simulink model "testemplanner_cs_old"  (R2020a)
settings: Solver=ode5  StartTime=0.0  StopTime=120  FixedStep=1/1000  RelTol=1e-3
PreLoadFcn:
  | mbxruntime.callbacks.PreLoadFcn(bdroot);
PostLoadFcn:
  | mbxruntime.callbacks.PostLoadFcn(bdroot);
InitFcn:
  | mbxruntime.callbacks.InitFcn(bdroot);
StartFcn:
  | mbxruntime.callbacks.StartFcn(bdroot);
StopFcn:
  | mbxruntime.callbacks.StopFcn(bdroot);
model workspace (MAT data in the model file):
  mbox_table : object (value not decoded)
  model_closed = 0
  sim_status = 0
values from neighbouring files (symbols this model uses):
  c_factor = 43.75    [emplanner_init.m]
  cf = -175016    [emplanner_init.m]
  cr = -130634    [emplanner_init.m]
  global_path_x = [0.057304 1.05668625507 2.05480936558 3.05165624935 4.04722112279 5.04150235808 6.03449985569 7.02621407764 8.01664569183 9.00579544113 9.99366409523 10.9802524329 ... (3001 elements, 3001x1)]    [global_path.mat]
  global_path_y = [8.29 8.29 8.29 8.29 8.29 8.29 8.29 8.29 8.29 8.29 8.29 8.29 ... (3001 elements, 3001x1)]    [global_path.mat]
  KD_PID_distance = 0.0    (= 0)    [emplanner_init.m]
  KD_PID_speed = 0    [emplanner_init.m]
  KI_PID_distance = 0.0    (= 0)    [emplanner_init.m]
  KI_PID_speed = 0    [emplanner_init.m]
  KP_PID_distance = 0.5    [emplanner_init.m]
  KP_PID_speed = 1.8    [emplanner_init.m]
  la = 1.265    [emplanner_init.m]
  lb = 2.947-1.265    (= 1.682)    [emplanner_init.m]
  LQR_K1 = k(:,1)'    [emplanner_init.m]
  LQR_K2 = k(:,2)'    [emplanner_init.m]
  LQR_K3 = k(:,3)'    [emplanner_init.m]
  LQR_K4 = k(:,4)'    [emplanner_init.m]
  m = 2020    [emplanner_init.m]
  rack_displacement = [-39.14 , -37.2 , -35.29 , -33.43 , -31.6 , -29.81 , -28.06 , -26.34 , -24.66 ,      -23.01 , -21.38 , -19.79 , -18.23 , -16.69 , -15.18 , -13.7 , -12.23 , -10.8 , -9.38 , -7.98 ,     -6.61 , -5.25 , -3.91 , -2.59 , -1.29 , 0 , 1.27 , 2.54 , 3.78 , 5.02 , 6.24 , 7.46 , 8.66 ,      9.86 , 11.05 , 12.24 , 13.41 , 14.59 , 15.76 , 16.92 , 18.09 , 19.25 , 20.42 , 21.59 , 22.76 ,      23.93 , 25.11 , 26 ...(+26 chars)    [emplanner_init.m]
  right_wheel_ground = [-70 ,-67.2 , -64.4 , -61.6 , -58.8 , -56 , -53.2 , -50.4 , -47.6 , -44.8 , -42 ,      -39.2 , -36.4 , -33.6 , -30.8 , -28 , -25.2 , -22.4 , -19.6 , -16.8 , -14 , -11.2 , -8.4 , -5.6 ,      -2.8 , 0 , 2.8 , 5.6 , 8.4 , 11.2 , 14 , 16.8 , 19.6 , 22.4 , 25.2 , 28 , 30.8 , 33.6 , 36.4 ,      39.2 , 42 , 44.8 , 47.6 , 50.4 , 53.2 , 56 , 58.8 , 61.6 , 64.4 , 67.2 , 70 ]    [emplanner_init.m]
  vx_break_point = zeros(1,5000)    [emplanner_init.m]
undefined symbols (not defined in the file or in its folder): aubr, DiscIntNeverNeededParam, tablebr, vubr
libraries: PreScanSimulinkLibrary x9, Solver_SF x1, simulink_extras x1
(part 4 of 6)

== system testemplanner_cs_old/Audi_A8_Sedan_1/Trajectories/Traj2State1/Traj2State2/Traj2MuxState_Ext ==
  Traj : Inport
  Terminator{1..9} (9 alike) : Terminator
  demux : Subsystem
  x [m] : Outport
  y [m] : Outport  Port=2
  z [m] : Outport  Port=3
  dx [m/s] : Outport  Port=4
  dy [m/s] : Outport  Port=5
  dz [m/s] : Outport  Port=6
  R [rad] : Outport  Port=7
  P [rad] : Outport  Port=8
  Y [rad] : Outport  Port=9
  wires:
  demux/9(Y) -> Y [rad]/1
  demux/7(R) -> R [rad]/1
  demux/5(vely) -> dy [m/s]/1
  demux/4(velx) -> dx [m/s]/1
  demux/10(velR) -> Terminator4/1
  demux/11(velP) -> Terminator5/1
  demux/12(velY) -> Terminator1/1
  demux/13(accx) -> Terminator8/1
  demux/14(accy) -> Terminator9/1
  demux/15(accz) -> Terminator7/1
  demux/18(accY) -> Terminator2/1
  demux/16(accR) -> Terminator3/1
  demux/17(accP) -> Terminator6/1
  demux/3(z) -> z [m]/1
  Traj/1 -> demux/1(traj)
  demux/6(velz) -> dz [m/s]/1
  demux/1(x) -> x [m]/1
  demux/2(y) -> y [m]/1
  demux/8(P) -> P [rad]/1

== system testemplanner_cs_old/Audi_A8_Sedan_1/control module1/control main/longitudinal control double PID/discrete pid ==
  err : Inport
  kp : Inport  Port=2
  ki : Inport  Port=3
  kd : Inport  Port=4
  Add2 : Sum  Inputs=+++
  Add3 : Sum
  Add4 : Sum  Inputs=+-
  Delay3 : Delay  DelayLength=1
  Delay4 : Delay  DelayLength=1
  Divide : Product  Inputs=**
  Divide1 : Product  Inputs=**
  Divide2 : Product  Inputs=**
  Gain : Gain  Gain=0.01
  pid_out : Outport
  wires:
  [KD_PID_distance] -> Divide2/2
  err/1 -> Delay4/1, Divide/2, Add3/1, Add4/1
  Divide/1 -> Add2/1
  Divide2/1 -> Add2/3
  Add3/1 -> Gain/1, Divide1/1
  Delay4/1 -> Add4/2
  [KP_PID_distance] -> Divide/1
  Divide1/1 -> Add2/2
  Delay3/1 -> Add3/2
  [KI_PID_distance] -> Divide1/2
  Add4/1 -> Divide2/1
  Add2/1 -> pid_out/1
  kp/1 -> [KP_PID_distance]
  ki/1 -> [KI_PID_distance]
  kd/1 -> [KD_PID_distance]
  Gain/1 -> Delay3/1

== system testemplanner_cs_old/Audi_A8_Sedan_1/control module1/control main/longitudinal control double PID/discrete pid1 ==
  err : Inport
  kp : Inport  Port=2
  ki : Inport  Port=3
  kd : Inport  Port=4
  Add2 : Sum  Inputs=+++
  Add3 : Sum
  Add4 : Sum  Inputs=+-
  Delay3 : Delay  DelayLength=1
  Delay4 : Delay  DelayLength=1
  Divide : Product  Inputs=**
  Divide1 : Product  Inputs=**
  Divide2 : Product  Inputs=**
  Gain : Gain  Gain=0.01
  pid_out : Outport
  wires:
  Gain/1 -> Delay3/1
  kd/1 -> [KD_PID_distance]
  ki/1 -> [KI_PID_distance]
  kp/1 -> [KP_PID_distance]
  Add2/1 -> pid_out/1
  Add4/1 -> Divide2/1
  [KI_PID_distance] -> Divide1/2
  Delay3/1 -> Add3/2
  Divide1/1 -> Add2/2
  [KP_PID_distance] -> Divide/1
  Delay4/1 -> Add4/2
  Add3/1 -> Divide1/1, Gain/1
  Divide2/1 -> Add2/3
  Divide/1 -> Add2/1
  err/1 -> Add4/1, Add3/1, Divide/2, Delay4/1
  [KD_PID_distance] -> Divide2/2

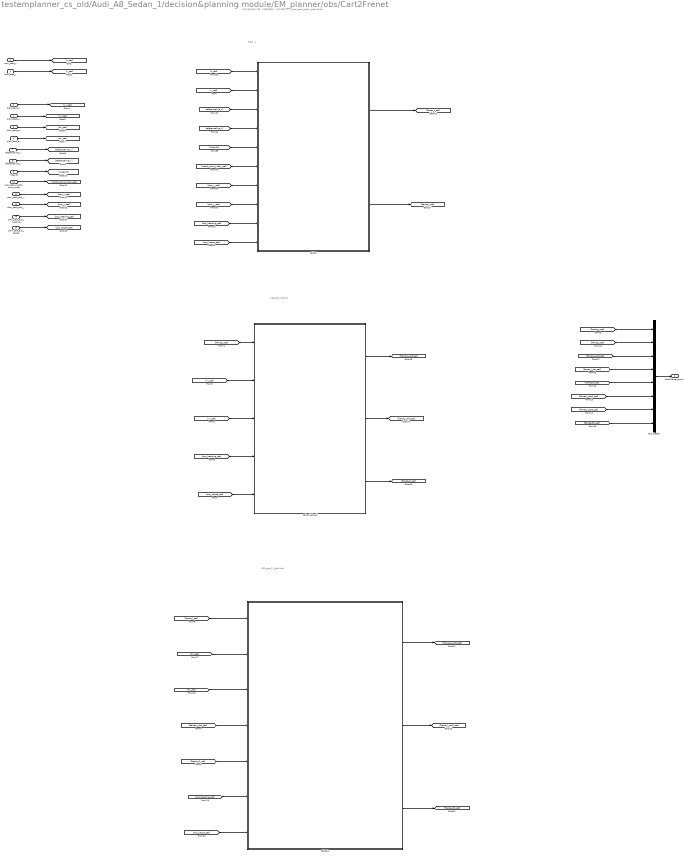
== system testemplanner_cs_old/Audi_A8_Sedan_1/decision&planning module/EM_planner/obs/Cart2Frenet ==
  note: 分成三部分进行计算，方便后续拆分，分别计算S，L，s_dot,l_dot,s_dot2,l_dot2,dl和ddl
  note: 计算S，L
  note: 计算s_dot,l_dot,dl
  note: 计算s_dot_2,l_dot2,ddl
  plan_start_x : Inport
  plan_start_y : Inport  Port=2
  plan_start_vx : Inport  Port=3
  plan_start_vy : Inport  Port=4
  plan_start_ax : Inport  Port=5
  plan_start_ay : Inport  Port=6
  referenceline_x : Inport  Port=7
  referenceline_y : Inport  Port=8
  index2s : Inport  Port=9
  plan_start_match_point_index : Inport  Port=10
  plan_start_proj_x : Inport  Port=11
  plan_start_proj_y : Inport  Port=12
  plan_start_proj_heading : Inport  Port=13
  plan_start_proj_kappa : Inport  Port=14
  Bus Creator : BusCreator  Inputs=8
  CalcSL : MATLAB Function  TreatAsAtomicUnit=on
  CalcSL2 : MATLAB Function  TreatAsAtomicUnit=on
  Calcs_l_dot_dl : MATLAB Function  TreatAsAtomicUnit=on
  Cart2Frenet_result : Outport
  wires:
  CalcSL/1(frenet_s_set) -> [frenet_s_set]
  plan_start_x/1 -> [x_set]
  plan_start_y/1 -> [y_set]
  plan_start_vx/1 -> [vx_set]
  plan_start_vy/1 -> [vy_set]
  plan_start_ax/1 -> [ax_set]
  plan_start_ay/1 -> [ay_set]
  referenceline_x/1 -> [referenceline_x]
  referenceline_y/1 -> [referenceline_y]
  index2s/1 -> [index2s]
  plan_start_match_point_index/1 -> [match_point_index_set]
  plan_start_proj_x/1 -> [proj_x_set]
  plan_start_proj_y/1 -> [proj_y_set]
  plan_start_proj_heading/1 -> [proj_heading_set]
  plan_start_proj_kappa/1 -> [proj_kappa_set]
  [x_set] -> CalcSL/1(x_set)
  [y_set] -> CalcSL/2(y_set)
  [referenceline_x] -> CalcSL/3(referenceline_x)
  [referenceline_y] -> CalcSL/4(referenceline_y)
  [index2s] -> CalcSL/5(index2s)
  [match_point_index_set] -> CalcSL/6(plan_start_match_point_index)
  [proj_x_set] -> CalcSL/7(plan_start_proj_x)
  [proj_y_set] -> CalcSL/8(plan_start_proj_y)
  [proj_heading_set] -> CalcSL/9(plan_start_proj_heading)
  [proj_kappa_set] -> CalcSL/10(plan_start_proj_kappa)
  [proj_kappa_set] -> Calcs_l_dot_dl/5(plan_start_proj_kappa)
  [proj_heading_set] -> Calcs_l_dot_dl/4(plan_start_proj_heading)
  [vx_set] -> Calcs_l_dot_dl/2(vx_set)
  [proj_heading_set] -> CalcSL2/6(plan_start_proj_heading)
  [proj_kappa_set] -> CalcSL2/7(plan_start_proj_kappa)
  CalcSL/2(frenet_l_set) -> [frenet_l_set]
  [frenet_l_set] -> Calcs_l_dot_dl/1(frenet_l_set)
  [vy_set] -> Calcs_l_dot_dl/3(vy_set)
  Calcs_l_dot_dl/1(s_dot_set) -> [frenet_s_dot_set]
  Calcs_l_dot_dl/2(l_dot_set) -> [frenet_l_dot_set]
  Calcs_l_dot_dl/3(dl_set) -> [frenet_dl_set]
  [ax_set] -> CalcSL2/2(ax_set)
  [ay_set] -> CalcSL2/3(ay_set)
  [frenet_dl_set] -> CalcSL2/5(dl_set)
  [frenet_l_set] -> CalcSL2/1(frenet_l_set)
  [frenet_s_dot_set] -> CalcSL2/4(s_dot_set)
  CalcSL2/3(ddl_set) -> [frenet_ddl_set]
  CalcSL2/2(l_dot2_set) -> [frenet_l_dot2_set]
  CalcSL2/1(s_dot2_set) -> [frenet_s_dot2_set]
  [frenet_s_set] -> Bus Creator/1
  [frenet_l_set] -> Bus Creator/2
  [frenet_s_dot_set] -> Bus Creator/3
  [frenet_l_dot_set] -> Bus Creator/4
  [frenet_dl_set] -> Bus Creator/5
  [frenet_s_dot2_set] -> Bus Creator/6
  [frenet_l_dot2_set] -> Bus Creator/7
  [frenet_ddl_set] -> Bus Creator/8
  Bus Creator/1 -> Cart2Frenet_result/1

== system testemplanner_cs_old/Audi_A8_Sedan_1/Trajectories/Traj2State1/Traj2State2/Traj2MuxState_Ext/demux ==
  traj : Inport
  Demux : Demux  Outputs=18
  x : Outport
  y : Outport  Port=2
  z : Outport  Port=3
  velx : Outport  Port=4
  vely : Outport  Port=5
  velz : Outport  Port=6
  R : Outport  Port=7
  P : Outport  Port=8
  Y : Outport  Port=9
  velR : Outport  Port=10
  velP : Outport  Port=11
  velY : Outport  Port=12
  accx : Outport  Port=13
  accy : Outport  Port=14
  accz : Outport  Port=15
  accR : Outport  Port=16
  accP : Outport  Port=17
  accY : Outport  Port=18
  wires:
  Demux/18 -> accY/1
  Demux/17 -> accP/1
  Demux/16 -> accR/1
  Demux/15 -> accz/1
  Demux/14 -> accy/1
  Demux/13 -> accx/1
  Demux/12 -> velY/1
  Demux/11 -> velP/1
  Demux/10 -> velR/1
  Demux/9 -> velz/1
  Demux/8 -> vely/1
  Demux/7 -> velx/1
  Demux/6 -> Y/1
  Demux/5 -> P/1
  traj/1 -> Demux/1
  Demux/4 -> R/1
  Demux/3 -> z/1
  Demux/2 -> y/1
  Demux/1 -> x/1

== matlab function testemplanner_cs_old/Audi_A8_Sedan_1/decision&planning module/EM_planner/Cart2Frenet/CalcSL ==
  data: x_set input; y_set input; referenceline_x input; referenceline_y input; index2s input; plan_start_match_point_index input; plan_start_proj_x input; plan_start_proj_y input; plan_start_proj_heading input; plan_start_proj_kappa input; frenet_s_set output; frenet_l_set output
function [frenet_s_set,frenet_l_set] =fcn(x_set,y_set,referenceline_x,referenceline_y,index2s,plan_start_match_point_index,plan_start_proj_x,plan_start_proj_y,plan_start_proj_heading,plan_start_proj_kappa)
%作用：这是一个通用函数，计算输入的笛卡尔坐标点x,y在自然坐标（frenet）坐标系中的s和l
%输入:要计算的点集的x,y坐标，航向，曲率。他的投影点的x,y坐标，index2s数据，以及参考线数据
%输出：自然坐标系下的s和l
%首先对s和l做一个缓冲
frenet_s_set=ones(128,1)*nan;
frenet_l_set=ones(128,1)*nan;
%开始计算
for i=1:length(x_set)
if isnan(x_set(i))  %遇到空的跳出
    break;
end
%调用相关函数进行s的计算
frenet_s_set(i)=CalcSfromIndex(referenceline_x,referenceline_y,plan_start_proj_x(i),plan_start_proj_y(i),plan_start_match_point_index(i),index2s);

%进行l的计算
%先求自然坐标系的切向量和法向量
%切向量,没用到
%tor=[cos(plan_start_proj_heading(i));sin(plan_start_proj_heading(i))];
%法向量
nor=[-sin(plan_start_proj_heading(i));cos(plan_start_proj_heading(i))];
frenet_l_set(i)=[x_set(i)-plan_start_proj_x(i);y_set(i)-plan_start_proj_y(i)]'*nor;
end

end
function s=CalcSfromIndex(ref_path_x,ref_path_y,match_point_x,match_point_y,match_point_index,index2s)   %使用一个函数来计算index所对应的S值
%%首先判断原点是在匹配点前还是匹配点后，通过向量的内积来进行判断
s_temp =  index2s(match_point_index);
vector1=[match_point_x-ref_path_x(match_point_index);match_point_y-ref_path_y(match_point_index)];
%考虑匹配点在路径终点的情况，不在终点就是匹配点和下一个点作为方向向量，如果是终点则使用匹配点和上一个点作为方向向量
if match_point_index<length(ref_path_x)
    vector2=[ref_path_x(match_point_index+1)-ref_path_x(match_point_index);ref_path_y(match_point_index+1)-ref_path_y(match_point_index)];
else
     vector2=[ref_path_x(match_point_index)-ref_path_x(match_point_index-1);ref_path_y(match_point_index)-ref_path_y(match_point_index-1)];
end
result=vector1'*vector2;    
if result >0 %原点在匹配点后，加上这个距离
    s=s_temp+sqrt(vector1'*vector1);
else        %原点在匹配点前，减去这个距离
    s=s_temp-sqrt(vector1'*vector1);
end
end

== matlab function testemplanner_cs_old/Audi_A8_Sedan_1/decision&planning module/EM_planner/Cart2Frenet/Calcs_l_dot_dl ==
  data: frenet_l_set input; vx_set input; vy_set input; plan_start_proj_heading input; plan_start_proj_kappa input; s_dot_set output; l_dot_set output; dl_set output
function [ s_dot_set, l_dot_set,dl_set]=fcn(frenet_l_set,vx_set,vy_set,plan_start_proj_heading,plan_start_proj_kappa)
%作用：通过之前计算得到的s和l值以及计算的速度值，计算s_dot,l_dot,以及dl
 %首先做一个缓冲
 n=128;
 s_dot_set=ones(n,1)*nan;
 l_dot_set=ones(n,1)*nan;
 dl_set=ones(n,1)*nan;

 for i=1:length(frenet_l_set)
     if isnan(frenet_l_set(i))
         break;
     end
    %先求自然坐标系的切向量和法向量
%切向量
tor=[cos(plan_start_proj_heading(i));sin(plan_start_proj_heading(i))];
%法向量
nor=[-sin(plan_start_proj_heading(i));cos(plan_start_proj_heading(i))];

vh=[vx_set(i);vy_set(i)];
l_dot_set(i)=vh'*nor;
s_dot_set(i)=vh'*tor/(1-plan_start_proj_kappa(i)*frenet_l_set(i));

if abs(s_dot_set(i))<1e-6
    dl_set(i)=0;
else
    dl_set(i)=l_dot_set(i)/s_dot_set(i);
 end
end

== matlab function testemplanner_cs_old/Audi_A8_Sedan_1/decision&planning module/EM_planner/Cart2Frenet/CalcSL2 ==
  data: frenet_l_set input; ax_set input; ay_set input; s_dot_set input; dl_set input; plan_start_proj_heading input; plan_start_proj_kappa input; s_dot2_set output; l_dot2_set output; ddl_set output
function [ s_dot2_set, l_dot2_set,ddl_set]=fcn(frenet_l_set,ax_set,ay_set,s_dot_set,dl_set,plan_start_proj_heading,plan_start_proj_kappa)
%作用：通过之前计算得到的l，s_dot、dl值以及已知的ax，ay值，计算s_dot2,l_dot2,以及ddl
 %首先做一个缓冲
 n=128;
 s_dot2_set=ones(n,1)*nan;
 l_dot2_set=ones(n,1)*nan;
 ddl_set=ones(n,1)*nan;

 for i=1:length(frenet_l_set)
     if isnan(frenet_l_set(i))
         break;
     end
    %先求自然坐标系的切向量和法向量
%切向量
tor=[cos(plan_start_proj_heading(i));sin(plan_start_proj_heading(i))];
%法向量
nor=[-sin(plan_start_proj_heading(i));cos(plan_start_proj_heading(i))];

ah=[ax_set(i);ay_set(i)];
l_dot2_set(i)=ah'*nor- plan_start_proj_kappa(i) * (1 - plan_start_proj_kappa(i) * frenet_l_set(i)) * s_dot_set(i)^2;
s_dot2_set(i)=(1/(1 - plan_start_proj_kappa(i) * frenet_l_set(i)))* (ah' * tor + 2 * plan_start_proj_kappa(i) * dl_set(i) * s_dot_set(i)^2);

if abs(s_dot2_set(i))<1e-6
    ddl_set(i)=0;
else
    ddl_set(i)=(l_dot2_set(i) - dl_set(i)*s_dot2_set(i))/(s_dot_set(i)^2);
 end
end

== matlab function testemplanner_cs_old/Audi_A8_Sedan_1/decision&planning module/referenceline provider/calc path heading and kappa ==
  data: path_x input; path_heading output; path_y input; path_kappa output
function [path_heading,path_kappa] = fcn(path_x,path_y)
%%函数，已知路径的坐标点，计算路径的航向角和曲率
dx=diff(path_x);
dy=diff(path_y);
path_heading_init1=atan2(dy,dx);
for i=1:length(path_heading_init1)
    if path_heading_init1(i)<0
        path_heading_init1(i)=path_heading_init1(i)+2*pi;
    end
end
path_heading=[path_heading_init1;path_heading_init1(end)];
d_heading=sin(diff(path_heading));

ds=sqrt(dx.^2+dy.^2);

path_kappa1=d_heading./ds;
path_kappa=[path_kappa1;path_kappa1(end)];

== matlab function testemplanner_cs_old/Audi_A8_Sedan_1/decision&planning module/EM_planner/obs/obs_fliter ==
  data: host_x input; obs_x_set_gcs_afterfliter output; host_y input; host_heading_xy input; obs_x_set_gcs input; obs_y_set_gcs input; obs_velocity_set_gcs input; obs_heading_set_gcs input; obs_y_set_gcs_afterfliter output; obs_velocity_set_gcs_afterfliter output; obs_heading_set_gcs_afterfliter output
function [obs_x_set_gcs_afterfliter,obs_y_set_gcs_afterfliter,obs_velocity_set_gcs_afterfliter,obs_heading_set_gcs_afterfliter] = fcn(host_x,host_y,host_heading_xy,obs_x_set_gcs,obs_y_set_gcs,obs_velocity_set_gcs,obs_heading_set_gcs)
%%作用：进行障碍筛选，只有在车辆纵向距离为[-10,60],横向距离为[-10，10]的障碍物才被处理
%%输入：车辆的坐标和航向，障碍物的坐标、速度和航向
%%输出：经过筛选后的障碍物的坐标、速度和航向

%%首先做一个缓冲
n=32; %只使用32个障碍物
obs_x_set_gcs_afterfliter=ones(n,1)*nan;
obs_y_set_gcs_afterfliter=ones(n,1)*nan;
obs_velocity_set_gcs_afterfliter=ones(n,1)*nan;
obs_heading_set_gcs_afterfliter=ones(n,1)*nan;
count=1;
%%
for i=1:length(obs_x_set_gcs)
    if isnan(obs_x_set_gcs(i))
        break;
    end
      %先求车辆坐标系的切向量和法向量
%切向量
tor=[cos(host_heading_xy(i));sin(host_heading_xy(i))];
%法向量
nor=[-sin(host_heading_xy(i));cos(host_heading_xy(i))];

lon_distance = [obs_x_set_gcs(i)-host_x;obs_y_set_gcs(i)-host_y]'*tor;
lat_distance = [obs_x_set_gcs(i)-host_x;obs_y_set_gcs(i)-host_y]'*nor;

if lon_distance>=-10 && lon_distance<=60&&lat_distance>=-10 && lat_distance<=10
    obs_x_set_gcs_afterfliter(count)=obs_x_set_gcs(i);
    obs_y_set_gcs_afterfliter(count)=obs_y_set_gcs(i);
    obs_velocity_set_gcs_afterfliter(count)=obs_velocity_set_gcs(i);
    obs_heading_set_gcs_afterfliter(count)=obs_heading_set_gcs(i);
    count=count+1;
end
end

== matlab function testemplanner_cs_old/Audi_A8_Sedan_1/decision&planning module/EM_planner/obs/obs_fliter_for_static ==
  data: obs_x_set_gcs_afterfliter input; obs_x_set_gcs_static output; obs_y_set_gcs_afterfliter input; obs_velocity_set_gcs_afterfliter input; obs_heading_set_gcs_afterfliter input; obs_y_set_gcs_static output; obs_x_set_gcs_dynamic output; obs_y_set_gcs_dynamic output; obs_velocity_set_gcs_dynamic output; obs_heading_set_gcs_dynamic output
function [obs_x_set_gcs_static,obs_y_set_gcs_static,obs_x_set_gcs_dynamic,obs_y_set_gcs_dynamic,obs_velocity_set_gcs_dynamic,obs_heading_set_gcs_dynamic] = fcn(obs_x_set_gcs_afterfliter,obs_y_set_gcs_afterfliter,obs_velocity_set_gcs_afterfliter,obs_heading_set_gcs_afterfliter)
%%作用：进行障碍筛选，只有在车辆纵向距离为[-10,60],横向距离为[-10，10]的障碍物才被处理
%%输入：车辆的坐标和航向，障碍物的坐标、速度和航向
%%输出：经过筛选后的障碍物的坐标、速度和航向

%%首先做一个缓冲
n=32; %只使用32个障碍物
obs_x_set_gcs_static=ones(n,1)*nan;
obs_y_set_gcs_static=ones(n,1)*nan;
obs_x_set_gcs_dynamic=ones(n,1)*nan;
obs_y_set_gcs_dynamic=ones(n,1)*nan;
obs_velocity_set_gcs_dynamic=ones(n,1)*nan;
obs_heading_set_gcs_dynamic=ones(n,1)*nan;
count_static=1;
count_dynamic=1;
%%
for i=1:length(obs_x_set_gcs_afterfliter)
   
if abs(obs_velocity_set_gcs_afterfliter)<0.1
    obs_x_set_gcs_static(count_static)=obs_x_set_gcs_afterfliter(i);
    obs_y_set_gcs_static(count_static)=obs_y_set_gcs_afterfliter(i);
    count_static=count_static+1;
else
    obs_x_set_gcs_dynamic(count_dynamic)=obs_x_set_gcs_afterfliter(i);
    obs_y_set_gcs_dynamic(count_dynamic)=obs_y_set_gcs_afterfliter(i);
    obs_velocity_set_gcs_dynamic(count_dynamic)=obs_velocity_set_gcs_afterfliter(i)*cos(obs_heading_set_gcs_afterfliter(i));
    obs_heading_set_gcs_dynamic(count_dynamic)=obs_velocity_set_gcs_afterfliter(i)*sin(obs_heading_set_gcs_afterfliter(i));
    count_dynamic=count_dynamic+1;
end
end

== matlab function testemplanner_cs_old/Audi_A8_Sedan_1/decision&planning module/referenceline provider/generate referenceline from global path ==
  data: host_match_point_index input; referenceline_x_init output; path_x input; path_y input; referenceline_y_init output
function [referenceline_x_init,referenceline_y_init] = fcn(host_match_point_index,path_x,path_y)
%根据匹配点提取参考线
%往前取30个点，往后取150个点。
%如果不够的话进行补齐


host_match_point_index_init=host_match_point_index(1);%取匹配点的第一个元素作为匹配点的序号，适用于获得车辆投影点的情况
start_index=-1;%初始化参考线起始点位置序号
end_index=-1;%初始化参考线终点位置序号
%一般来讲从匹配点向前寻找30个点，向后寻找150个点。
if host_match_point_index_init< 31    %如果向前寻找的点不够30个，则选取最初的180个点
    start_index=1;
elseif host_match_point_index_init> length(path_x)-150 %如果向后寻找的点不够150个，则选取最后的180个点
    
    start_index=length(path_x)-180;
else                                                 %其他情况下则是向前选取30个点，向后选取150个点
    start_index=host_match_point_index_init-30;
    
end
referenceline_x_init=path_x(start_index:start_index+180);             %提取参考线x坐标
referenceline_y_init=path_y(start_index:start_index+180);             %提取参考线y坐标

== matlab function testemplanner_cs_old/Audi_A8_Sedan_1/decision&planning module/EM_planner/general fast algorithm to find projection point info2 ==
  data: x_set input; match_point_index_set output; y_set input; path_x input; path_y input; proj_x_set output; proj_y_set output; proj_heading_set output; proj_kappa_set output; path_heading input; path_kappa input
function [match_point_index_set,proj_x_set,proj_y_set,proj_heading_set,proj_kappa_set] = fcn(x_set,y_set,path_x,path_y,path_heading,path_kappa)
%该函数是一个通用函数，找到x_set,y_set在path_x,path_y的匹配点的编号，以及投影点在直角坐标系下的(x,y,theta,kappa)
%最多可以处理128个点

match_point_index_set = ones(128,1)*nan;
proj_x_set = ones(128,1)*nan;
proj_y_set = ones(128,1)*nan;
proj_heading_set = ones(128,1)*nan;
proj_kappa_set = ones(128,1)*nan;

persistent is_first_run;
persistent init_search_index_set;
persistent pre_frenet_path_x;
persistent pre_frenet_path_y;
persistent pre_frenet_path_heading;
persistent pre_frenet_path_kappa;
if isempty(is_first_run)
    is_first_run = 0; 
    init_search_index_set = ones(128,1)*nan;
    start_index = 1;
    pre_frenet_path_x = path_x;
    pre_frenet_path_y = path_y;
    pre_frenet_path_heading = path_heading;
    pre_frenet_path_kappa = path_kappa;
    for i = 1:length(x_set)
        if isnan(x_set(i))
            break;
        else
            increase_count = 0;
            min_distance = 1e10;
            for j = start_index:length(path_x)
                distance = (x_set(i)-path_x(j))^2 + (y_set(i)-path_y(j))^2;
                if (min_distance > distance)
                    min_distance = distance;
                    init_search_index_set(i)=j;
                    increase_count = 0;
                else
                    increase_count = increase_count + 1;
                end
                if increase_count > 50
                    break;
                end
            end
            match_point_index = init_search_index_set(i);
            match_point_index_set(i) = match_point_index;
            vector_match_point = [path_x(match_point_index);path_y(match_point_index)];
            vector_match_point_direction = [cos(path_heading(match_point_index));sin(path_heading(match_point_index))];
            vector_host_point = [x_set(i);y_set(i)];
            vector_d = vector_host_point - vector_match_point;
            vector_err = (vector_d'* vector_match_point_direction) * vector_match_point_direction;
            vector_proj = vector_err + vector_match_point;
            proj_x_set(i) = vector_proj(1);
            proj_y_set(i) = vector_proj(2);
            proj_heading_set(i) = path_heading(match_point_index) + path_kappa(match_point_index) * (vector_d'* vector_match_point_direction);
            proj_kappa_set(i) = path_kappa(match_point_index);            
        end
    end 
    init_search_index_set=match_point_index_set;
else
    min_distance = inf;
    for i = 1:length(x_set)
        increase_count = 0;
        count_limit=5;
        if isnan(init_search_index_set(i))
            start_index = 1;
            count_limit=50;
       
        
        else
            
            start_index = init_search_index_set(i);
          
         end  
            
            vector_m_init = [pre_frenet_path_x(start_index);pre_frenet_path_y(start_index)];
            vector_direction_init = [cos(pre_frenet_path_heading(start_index));sin(pre_frenet_path_heading(start_index))];
            ds = vector_m_init'*vector_direction_init;
            if ds > 0.001            
                for j = start_index:length(pre_frenet_path_x )
                    distance = (x_set(i)-pre_frenet_path_x (j))^2 + (y_set(i)-pre_frenet_path_y(j))^2;
                    if (min_distance > distance)
                        min_distance = distance;
                        init_search_index_set(i)=j;
                        increase_count = 0;
                    else
                        increase_count = increase_count + 1;
                    end
                    if increase_count > count_limit
                        break;
                    end
                end
            elseif ds < -0.001
                for j = start_index:-1:1
                    distance = (x_set(i)-pre_frenet_path_x (j))^2 + (y_set(i)-pre_frenet_path_y(j))^2;
                    if (min_distance > distance)
                        min_distance = distance;
                        init_search_index_set(i)=j;
                        increase_count = 0;
                    else
                        increase_count = increase_count + 1;
                    end
                    if increase_count >  count_limit
                        break;
                    end
                end
            end
            match_point_index = init_search_index_set(i);
            match_point_index_set(i) = match_point_index;
            vector_match_point = [pre_frenet_path_x(match_point_index);pre_frenet_path_y(match_point_index)];
            vector_match_point_direction = [cos(pre_frenet_path_heading(match_point_index));sin(pre_frenet_path_heading(match_point_index))];
            vector_host_point = [x_set(i);y_set(i)];
            vector_d = vector_host_point - vector_match_point;
            vector_err = (vector_d'* vector_match_point_direction) * vector_match_point_direction;
            vector_proj = vector_err + vector_match_point;
            proj_x_set(i) = vector_proj(1);
            proj_y_set(i) = vector_proj(2);
            proj_heading_set(i) = pre_frenet_path_heading(match_point_index) + pre_frenet_path_kappa(match_point_index) * (vector_d'* vector_match_point_direction);
            proj_kappa_set(i) = pre_frenet_path_kappa(match_point_index);            
        end
    end    
    init_search_index_set = match_point_index_set;
    pre_frenet_path_x = path_x;
    pre_frenet_path_y = path_y;
    pre_frenet_path_heading = path_heading;
    pre_frenet_path_kappa = path_kappa;
end

== matlab function testemplanner_cs_old/Audi_A8_Sedan_1/decision&planning module/referenceline provider/reference_line_smooth ==
  data: referenceline_x_init input; referenceline_x output; referenceline_y_init input; pre_referenceline_x input; pre_referenceline_y input; w_ref_cost input; w_smooth_cost input; w_length_cost input; referenceline_x_lb input; referenceline_x_ub input; referenceline_y_lb input; referenceline_y_ub input; referenceline_y output
function [referenceline_x,referenceline_y] = fcn(referenceline_x_init,referenceline_y_init,pre_referenceline_x,pre_referenceline_y,w_ref_cost,w_smooth_cost,w_length_cost,referenceline_x_lb,referenceline_x_ub,referenceline_y_lb,referenceline_y_ub)
coder.extrinsic('quadprog');
%%此函数功能是利用二次规划的方法进行参考线的平滑

%输入：原始参考线点集
%输出：平滑后的参考线点集
%cost function =
%w1*((xi-xiref)^2+(yi-yiref)^2)+w2*((x（i-1）+x（i+1）-2xi)^2+(y（i-1）+y（i+1）-2yi)^2)+w3*((x（i+1）-xi)^2+(y（i+1）-yi)^2)

%首先确定数据维数
n=181;
persistent is_first_run
persistent pre_reference_x
persistent pre_reference_y
 
% if isempty(is_first_run)
%     is_first_run=0;
% %根据二次规划 1/2x'Hx+f'x=min
% %                Ax<=b
%  %               lb=<x,+yb
%  
%  %首先定义矩阵A1,A2,A3
%  A1=zeros(2*n-4,2*n);%平滑代价系数矩阵
%  A2=zeros(2*n-2,2*n);%紧凑代价系数矩阵
%  A3=eye(2*n,2*n);%几何相似代价系数矩阵
%  
%  M=zeros(2*n,1);
%  lb=M;
%  ub=M;
%  for i=1:n
%      M(2*i-1)=reference_line_x_init(i);
%      M(2*i)=reference_line_y_init(i);
%      lb(2*i-1)=reference_line_x_init(i)+reference_line_x_lb;
%      lb(2*i)=reference_line_y_init(i)+reference_line_y_lb;
%      ub(2*i-1)=reference_line_x_ub+reference_line_x_init(i);
%      ub(2*i)=reference_line_y_ub+reference_line_y_init(i);
%  end
% 
%  for j=1:2:2*n-5
%      A1(j,j)=1;
%      A1(j,j+2)=-2;
%      A1(j,j+4)=1;
%      A1(j+1,j+1)=1;
%      A1(j+1,j+3)=-2;
%      A1(j+1,j+5)=1;
%  end
%   for k=1:2:2*n-3
%      A2(k,k)=1;
%      A2(k,k+2)=-1;
%      A2(k+1,k+1)=1;
%      A2(k+1,k+3)=-1;
%   end
% H=w_smooth_cost*(A1'*A1)+w_length_cost*(A2'*A2)+w_ref_cost*A3; 
% H = 2 * H;
% X0 = M;
% f = -2*w_ref_cost*M;
if isempty(is_first_run)
    is_first_run = 0;
    A1=zeros(2*n-4,2*n);
    A2=zeros(2*n-2,2*n);
    f=zeros(n*2,1);
    lb=f;
    ub=f;
    for i=1:n
    f(2*i-1)=referenceline_x_init(i);
    f(2*i)=referenceline_y_init(i);
    lb(2*i-1)=referenceline_x_init(i)+referenceline_x_lb;
    lb(2*i)=referenceline_y_init(i)+referenceline_y_lb;
    ub(2*i-1)=referenceline_x_init(i)+referenceline_x_ub;
    ub(2*i)=referenceline_y_init(i)+referenceline_y_ub;
    end

    for i=1:2:2*n-5
    A1(i,i)=1;
    A1(i,i+2)=-2;
    A1(i,i+4)=1;
    A1(i+1,i+1)=1;
    A1(i+1,i+3)=-2;
    A1(i+1,i+5)=1; 
    end
    for i=1:2:2*n-3
    A2(i,i)=1;
    A2(i,i+2)=-1;    
    A2(i+1,i+1)=1;
    A2(i+1,i+3)=-1;  
    end
    A3=eye(2*n,2*n);
    H=w_smooth_cost*(A1'*A1)+w_length_cost*(A2'*A2)+w_ref_cost*A3;
    H=2*H;
    X0=f;
    f=-2*w_ref_cost*f;
    X=quadprog(H,f,[],[],[],[],lb,ub,X0);
    
%     x=zeros(n,1);
%     y=zeros(n,1);
%     for i=1:n
%         x(i)=X(2*i-1);
%         y(i)=X(2*i);
%     end
%     if isempty(is_first_run)
%     is_first_run = 0;
%     A1=zeros(2*n-4,2*n);
%     A2=zeros(2*n-2,2*n);
%     f=zeros(n*2,1);
%     lb=f;
%     ub=f;
%     for i=1:n
%     f(2*i-1)=referenceline_x_init(i);
%     f(2*i)=referenceline_y_init(i);
%     lb(2*i-1)=referenceline_x_init(i)+referenceline_x_lb;
%     lb(2*i)=referenceline_y_init(i)+referenceline_y_lb;
%     ub(2*i-1)=referenceline_x_init(i)+referenceline_x_ub;
%     ub(2*i)=referenceline_y_init(i)+referenceline_y_ub;
%     end

%     for i=1:2:2*n-5
%     A1(i,i)=1;
%     A1(i,i+2)=-2;
%     A1(i,i+4)=1;
%     A1(i+1,i+1)=1;
%     A1(i+1,i+3)=-2;
%     A1(i+1,i+5)=1; 
%     end
%     for i=1:2:2*n-3
%     A2(i,i)=1;
%     A2(i,i+2)=-1;    
%     A2(i+1,i+1)=1;
%     A2(i+1,i+3)=-1;  
%     end
%     A3=eye(2*n,2*n);
%     H=w_smooth_cost*(A1'*A1)+w_length_cost*(A2'*A2)+w_ref_cost*A3;
%     H=2*H;
%     X0=f;
%     f=-2*w_ref_cost*f;

%     X=quadprog(H,f,[],[],[],[],lb,ub,X0);
    x=zeros(n,1);
    y=zeros(n,1);

    for i=1:n
    x(i)=X(2*i-1);
    y(i)=X(2*i);
    end
    referenceline_x=x;
    referenceline_y=y;
    pre_reference_x=x;
    pre_reference_y=y;
else
    index=-1;
    new_reference_line_x=referenceline_x_init(1);
    new_reference_line_y=referenceline_y_init(1);
    for i=1:length(pre_referenceline_x)
        if (pre_referenceline_x(i)==new_reference_line_x)&&(pre_referenceline_y(i)==new_reference_line_y)
            index=i;
            break;
        end
    end
        if index==-1||index>6
            %首先定义矩阵A1,A2,A3
            A1=zeros(2*n-4,2*n);%平滑代价系数矩阵
            A2=zeros(2*n-2,2*n);%紧凑代价系数矩阵
            A3=eye(2*n,2*n);%几何相似代价系数矩阵
            
            M=zeros(2*n,1);
            lb=M;
            ub=M;
            for i=1:n
                M(2*i-1)=referenceline_x_init(i);
                M(2*i)=referenceline_y_init(i);
                lb(2*i-1)=referenceline_x_init(i)-referenceline_x_lb;
                lb(2*i)=referenceline_y_init(i)-referenceline_y_lb;
                ub(2*i-1)=referenceline_x_ub+referenceline_x_init(i);
                ub(2*i)=referenceline_y_ub+referenceline_y_init(i);
            end
            
            for i=1:2:2*n-5
                A1(i,i)=1;
                A1(i,i+2)=-2;
                A1(i,i+4)=1;
                A1(i+1,i+1)=1;
                A1(i+1,i+3)=-2;
                A1(i+1,i+5)=1;
            end
            for i=1:2:2*n-3
                A2(i,i)=1;
                A2(i,i+2)=-1;
                A2(i+1,i+1)=1;
                A2(i+1,i+3)=-1;
            end
            H=2*(w_smooth_cost*(A1'*A1)+w_length_cost*(A2'*A2)+w_ref_cost*A3);
            f = w_ref_cost*(-2*M);
            X=quadprog(H,f,[],[],[],[],lb,ub,M);
            x=zeros(n,1);
            y=zeros(n,1);
            for i=1:n
                x(i)=X(2*i-1);
                y(i)=X(2*i);
            end
            referenceline_x=x;
            referenceline_y=y;
            pre_reference_x=x;
            pre_reference_y=y;
        elseif index==1
            referenceline_x=pre_reference_x;
            referenceline_y=pre_reference_y;   
        else
            %开始进行轨迹拼接，但是拼接点的个数无法确定，先定义成6个,但因为要带上原有轨迹的两个点，所以是6+2个
            point_num=6+2;
            A1=zeros(2*point_num-4,2*point_num);%平滑代价系数矩阵
            A2=zeros(2*point_num-2,2*point_num);%紧凑代价系数矩阵
            A3=eye(2*point_num,2*point_num);%几何相似代价系数矩阵
              
            M=zeros(2*point_num,1);
            lb=M;
            ub=M;
            
            %要拼接的点个数是序号-1
            joint_num=index-1;
            M(1)=pre_reference_x(length(referenceline_x_init) - 1);
            M(2)=pre_reference_y(length(referenceline_x_init) - 1);
            M(3)=pre_reference_x(length(referenceline_x_init));
            M(4)=pre_reference_y(length(referenceline_x_init));
            lb(1)=M(1);
            lb(2)=M(2);
            lb(3)=M(3);
            lb(4)=M(4);
            ub(1)=M(1);
            ub(2)=M(2);
            ub(3)=M(3);
            ub(4)=M(4);
            %因为前面有joint_num个点是一样的，所以只需要平滑最后剩下的几个点即可
            start_index=length(referenceline_x_init)-joint_num;
            for i=1:joint_num
            M(2*i+3)=referenceline_x_init(start_index+i);
            M(2*i+4)=referenceline_y_init(start_index+i);
            lb(2*i+3)=referenceline_x_init(start_index+i)-referenceline_x_lb;
            lb(2*i+4)=referenceline_y_init(start_index+i)-referenceline_y_lb;
            ub(2*i+3)=referenceline_x_init(start_index+i)+referenceline_x_ub;
            ub(2*i+4)=referenceline_y_init(start_index+i)+referenceline_y_ub;
            end
             for i=1:2:2*(joint_num+2)-5
                A1(i,i)=1;
                A1(i,i+2)=-2;
                A1(i,i+4)=1;
                A1(i+1,i+1)=1;
                A1(i+1,i+3)=-2;
                A1(i+1,i+5)=1;
            end
            for i=1:2:2*(joint_num+2)-3
                A2(i,i)=1;
                A2(i,i+2)=-1;
                A2(i+1,i+1)=1;
                A2(i+1,i+3)=-1;
            end
            H=2*(w_smooth_cost*(A1'*A1)+w_length_cost*(A2'*A2)+w_ref_cost*(A3'*A3));
            f = w_ref_cost*(-2*M);
            X=quadprog(H,f,[],[],[],[],lb,ub,M);
            x=zeros(joint_num,1);
            y=zeros(joint_num,1);
            for i=1:joint_num
                x(i)=X(2*i+3);
                y(i)=X(2*i+4);
            end
            referenceline_x=zeros(n,1);
            referenceline_y=zeros(n,1);
            %进行轨迹拼接
            for i=1:length(referenceline_x_init)
                if i<=length(referenceline_x_init)-joint_num
                    referenceline_x(i)=pre_reference_x(i+joint_num);
                    referenceline_y(i)=pre_reference_y(i+joint_num);
                else
                    referenceline_x(i)=x(i-length(referenceline_x_init)+joint_num);
                    referenceline_y(i)=y(i-length(referenceline_x_init)+joint_num);
                end
            end
            
            pre_reference_x=referenceline_x;
            pre_reference_y=referenceline_y;
         
        end
end

== matlab function testemplanner_cs_old/Audi_A8_Sedan_1/decision&planning module/EM_planner/obs/general fast algorithm to find projection point info1 ==
  data: x_set input; match_point_index_set output; y_set input; path_x input; path_y input; proj_x_set output; proj_y_set output; proj_heading_set output; proj_kappa_set output; path_heading input; path_kappa input
function [match_point_index_set,proj_x_set,proj_y_set,proj_heading_set,proj_kappa_set] = fcn(x_set,y_set,path_x,path_y,path_heading,path_kappa)
%该函数是一个通用函数，找到x_set,y_set在path_x,path_y的匹配点的编号，以及投影点在直角坐标系下的(x,y,theta,kappa)
%最多可以处理128个点

match_point_index_set = ones(128,1)*nan;
proj_x_set = ones(128,1)*nan;
proj_y_set = ones(128,1)*nan;
proj_heading_set = ones(128,1)*nan;
proj_kappa_set = ones(128,1)*nan;

persistent is_first_run;
persistent init_search_index_set;
persistent pre_frenet_path_x;
persistent pre_frenet_path_y;
persistent pre_frenet_path_heading;
persistent pre_frenet_path_kappa;
if isempty(is_first_run)
    is_first_run = 0; 
    init_search_index_set = ones(128,1)*nan;
    start_index = 1;
    pre_frenet_path_x = path_x;
    pre_frenet_path_y = path_y;
    pre_frenet_path_heading = path_heading;
    pre_frenet_path_kappa = path_kappa;
    for i = 1:length(x_set)
        if isnan(x_set(i))
            break;
        else
            increase_count = 0;
            min_distance = 1e10;
            for j = start_index:length(path_x)
                distance = (x_set(i)-path_x(j))^2 + (y_set(i)-path_y(j))^2;
                if (min_distance > distance)
                    min_distance = distance;
                    init_search_index_set(i)=j;
                    increase_count = 0;
                else
                    increase_count = increase_count + 1;
                end
                if increase_count > 50
                    break;
                end
            end
            match_point_index = init_search_index_set(i);
            match_point_index_set(i) = match_point_index;
            vector_match_point = [path_x(match_point_index);path_y(match_point_index)];
            vector_match_point_direction = [cos(path_heading(match_point_index));sin(path_heading(match_point_index))];
            vector_host_point = [x_set(i);y_set(i)];
            vector_d = vector_host_point - vector_match_point;
            vector_err = (vector_d'* vector_match_point_direction) * vector_match_point_direction;
            vector_proj = vector_err + vector_match_point;
            proj_x_set(i) = vector_proj(1);
            proj_y_set(i) = vector_proj(2);
            proj_heading_set(i) = path_heading(match_point_index) + path_kappa(match_point_index) * (vector_d'* vector_match_point_direction);
            proj_kappa_set(i) = path_kappa(match_point_index);            
        end
    end 
    init_search_index_set=match_point_index_set;
else
    min_distance = inf;
    for i = 1:length(x_set)
        increase_count = 0;
        count_limit=5;
        if isnan(init_search_index_set(i))
            start_index = 1;
            count_limit=50;
       
        
        else
            
            start_index = init_search_index_set(i);
          
         end  
            
            vector_m_init = [pre_frenet_path_x(start_index);pre_frenet_path_y(start_index)];
            vector_direction_init = [cos(pre_frenet_path_heading(start_index));sin(pre_frenet_path_heading(start_index))];
            ds = vector_m_init'*vector_direction_init;
            if ds > 0.001            
                for j = start_index:length(pre_frenet_path_x )
                    distance = (x_set(i)-pre_frenet_path_x (j))^2 + (y_set(i)-pre_frenet_path_y(j))^2;
                    if (min_distance > distance)
                        min_distance = distance;
                        init_search_index_set(i)=j;
                        increase_count = 0;
                    else
                        increase_count = increase_count + 1;
                    end
                    if increase_count > count_limit
                        break;
                    end
                end
            elseif ds < -0.001
                for j = start_index:-1:1
                    distance = (x_set(i)-pre_frenet_path_x (j))^2 + (y_set(i)-pre_frenet_path_y(j))^2;
                    if (min_distance > distance)
                        min_distance = distance;
                        init_search_index_set(i)=j;
                        increase_count = 0;
                    else
                        increase_count = increase_count + 1;
                    end
                    if increase_count >  count_limit
                        break;
                    end
                end
            end
            match_point_index = init_search_index_set(i);
            match_point_index_set(i) = match_point_index;
            vector_match_point = [pre_frenet_path_x(match_point_index);pre_frenet_path_y(match_point_index)];
            vector_match_point_direction = [cos(pre_frenet_path_heading(match_point_index));sin(pre_frenet_path_heading(match_point_index))];
            vector_host_point = [x_set(i);y_set(i)];
            vector_d = vector_host_point - vector_match_point;
            vector_err = (vector_d'* vector_match_point_direction) * vector_match_point_direction;
            vector_proj = vector_err + vector_match_point;
            proj_x_set(i) = vector_proj(1);
            proj_y_set(i) = vector_proj(2);
            proj_heading_set(i) = pre_frenet_path_heading(match_point_index) + pre_frenet_path_kappa(match_point_index) * (vector_d'* vector_match_point_direction);
            proj_kappa_set(i) = pre_frenet_path_kappa(match_point_index);            
        end
    end    
    init_search_index_set = match_point_index_set;
    pre_frenet_path_x = path_x;
    pre_frenet_path_y = path_y;
    pre_frenet_path_heading = path_heading;
    pre_frenet_path_kappa = path_kappa;
end

== matlab function testemplanner_cs_old/Audi_A8_Sedan_1/control module1/control main/chassic steering system/MATLAB Function ==
  data: u input; right_steer output; la input; lb input
function right_steer = fcn(u,la,lb)
if abs(u)<1e-2
   right_steer = u;
else
   R =  (la+lb)/tan(u);
   right_steer = atan((la+lb)/(R+1.624/2));
end

== matlab function testemplanner_cs_old/Audi_A8_Sedan_1/control module1/control main/lateral control LQR/calc lqr K ==
  data: k1 input; k output; k2 input; k3 input; k4 input; vx input
function k  = fcn(k1,k2,k3,k4,vx)
    if abs(vx)<0.1
        k=[0,0,0,0];
    else
       
        k=[k1,k2,k3,k4];
    end
end

== matlab function testemplanner_cs_old/Audi_A8_Sedan_1/control module1/control main/lateral control LQR/err_kappa_calculate_module ==
  data: x input; y input; phi input; vx input; vy input; phi_dot input; xr input; yr input; thetar input; kappar input; err output; es output; s_dot output; phi output; projection_point_thetar output
function [err,es,s_dot,phi,projection_point_thetar] = fcn(x,y,phi,vx,vy,phi_dot,xr,yr,thetar,kappar)
    
    tor=[cos(thetar);sin(thetar)];
    nor=[-sin(thetar);cos(thetar)];
    d_err=[x-xr;y-yr];
    ed=nor'*d_err;
    es=tor'*d_err;
    %projection_point_thetar=thetar(dmin);%apollo
    projection_point_thetar=thetar+kappar*es;
    ed_dot=vy*cos(phi-projection_point_thetar)+vx*sin(phi-projection_point_thetar);
    %%%%%%%%%
    ephi=sin(phi-projection_point_thetar);
    %%%%%%%%%
    ss_dot=vx*cos(phi-projection_point_thetar)-vy*sin(phi-projection_point_thetar);
    s_dot=ss_dot/(1-kappar*ed);
    ephi_dot=phi_dot-kappar*s_dot;
    err=[ed;ed_dot;ephi;ephi_dot];
    
    
    
    
    
    
    
    
    
    
    
    


end

== matlab function testemplanner_cs_old/Audi_A8_Sedan_1/control module1/control main/lateral control LQR/feed_forword_control ==
  data: vx input; a input; forword_angle output; b input; m input; cf input; cr input; k input; kr input
function forword_angle = fcn(vx,a,b,m,cf,cr,k,kr)
    forword_angle=kr*(a+b-b*k(3)-(m*vx*vx/(a+b))*((b/cf)+(a/cr)*k(3)-(a/cr)));
end

== matlab function testemplanner_cs_old/Audi_A8_Sedan_1/control module1/control main/lateral control LQR/feedback_control+feedforword_control ==
  data: k input; angle output; err input; forword_angle input
function angle = fcn(k,err,forword_angle)

    angle=-k*err+forword_angle;
end

== matlab function testemplanner_cs_old/Audi_A8_Sedan_1/control module1/control main/lateral control LQR/predict_module ==
  data: x input; pred_x_ctrl output; y input; phi input; vx input; vy input; phi_dot input; ts input; pred_y_ctrl output; pred_yaw_ctrl output; pred_vx_ctrl output; pred_vy_ctrl output; pred_yaw_dot_ctrl output
function [pred_x_ctrl,pred_y_ctrl,pred_yaw_ctrl,pred_vx_ctrl,pred_vy_ctrl,pred_yaw_dot_ctrl] = fcn(x,y,phi,vx,vy,phi_dot,ts)
    pred_x_ctrl=x+vx*ts*cos(phi)-vy*ts*sin(phi);
    pred_y_ctrl=y+vy*ts*cos(phi)+vx*ts*sin(phi);
    pred_yaw_ctrl=phi;
    pred_vx_ctrl=vx;
    pred_vy_ctrl=vy;
    pred_yaw_dot_ctrl=phi_dot;
end

== matlab function testemplanner_cs_old/Audi_A8_Sedan_1/control module1/control main/longitudinal control double PID/MATLAB Function1 ==
  data: u input; throttle output; brake output
function [throttle,brake] = fcn(u)
    if u>=0
        throttle=u;
        brake=0;
    else
        throttle=0;
        brake=-u;
    end

== matlab function testemplanner_cs_old/Audi_A8_Sedan_1/decision&planning module/EM_planner/obs/Cart2Frenet/CalcSL ==
  data: x_set input; y_set input; referenceline_x input; referenceline_y input; index2s input; plan_start_match_point_index input; plan_start_proj_x input; plan_start_proj_y input; plan_start_proj_heading input; plan_start_proj_kappa input; frenet_s_set output; frenet_l_set output
function [frenet_s_set,frenet_l_set] =fcn(x_set,y_set,referenceline_x,referenceline_y,index2s,plan_start_match_point_index,plan_start_proj_x,plan_start_proj_y,plan_start_proj_heading,plan_start_proj_kappa)
%作用：这是一个通用函数，计算输入的笛卡尔坐标点x,y在自然坐标（frenet）坐标系中的s和l
%输入:要计算的点集的x,y坐标，航向，曲率。他的投影点的x,y坐标，index2s数据，以及参考线数据
%输出：自然坐标系下的s和l
%首先对s和l做一个缓冲
frenet_s_set=ones(128,1)*nan;
frenet_l_set=ones(128,1)*nan;
%开始计算
for i=1:length(x_set)
if isnan(x_set(i))  %遇到空的跳出
    break;
end
%调用相关函数进行s的计算
frenet_s_set(i)=CalcSfromIndex(referenceline_x,referenceline_y,plan_start_proj_x(i),plan_start_proj_y(i),plan_start_match_point_index(i),index2s);

%进行l的计算
%先求自然坐标系的切向量和法向量
%切向量,没用到
%tor=[cos(plan_start_proj_heading(i));sin(plan_start_proj_heading(i))];
%法向量
nor=[-sin(plan_start_proj_heading(i));cos(plan_start_proj_heading(i))];
frenet_l_set(i)=[x_set(i)-plan_start_proj_x(i);y_set(i)-plan_start_proj_y(i)]'*nor;
end

end
function s=CalcSfromIndex(ref_path_x,ref_path_y,match_point_x,match_point_y,match_point_index,index2s)   %使用一个函数来计算index所对应的S值
%%首先判断原点是在匹配点前还是匹配点后，通过向量的内积来进行判断
s_temp =  index2s(match_point_index);
vector1=[match_point_x-ref_path_x(match_point_index);match_point_y-ref_path_y(match_point_index)];
%考虑匹配点在路径终点的情况，不在终点就是匹配点和下一个点作为方向向量，如果是终点则使用匹配点和上一个点作为方向向量
if match_point_index<length(ref_path_x)
    vector2=[ref_path_x(match_point_index+1)-ref_path_x(match_point_index);ref_path_y(match_point_index+1)-ref_path_y(match_point_index)];
else
     vector2=[ref_path_x(match_point_index)-ref_path_x(match_point_index-1);ref_path_y(match_point_index)-ref_path_y(match_point_index-1)];
end
result=vector1'*vector2;    
if result >0 %原点在匹配点后，加上这个距离
    s=s_temp+sqrt(vector1'*vector1);
else        %原点在匹配点前，减去这个距离
    s=s_temp-sqrt(vector1'*vector1);
end
end
